simulink model "untitled2021315"  (R2018b)
settings: Solver=VariableStepAuto  StartTime=0.0  StopTime=0.001  RelTol=1e-3
libraries: simulink x2
settings Model: Creator=zyh  LastModifiedBy=zyh

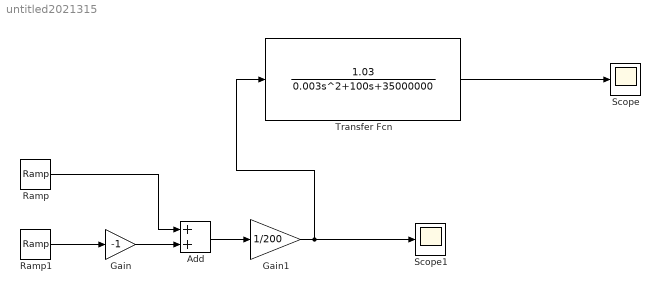
== system untitled2021315 ==
  Add : Sum
  Gain : Gain  Gain=-1
  Gain1 : Gain  Gain=1/200
  Ramp : simulink/Sources/Ramp  slope=600000000  start=0  InitialOutput=0
  Ramp1 : simulink/Sources/Ramp  slope=600000000  start=0.00005  InitialOutput=0
  Scope : Scope
  Scope1 : Scope
  Transfer Fcn : TransferFcn  Numerator=[1.03]  Denominator=[0.003 100 35000000]
  wires:
  Transfer Fcn/1 -> Scope/1
  Ramp1/1 -> Gain/1
  Gain/1 -> Add/2
  Ramp/1 -> Add/1
  Add/1 -> Gain1/1
  Gain1/1 -> Scope1/1, Transfer Fcn/1
